simulink library "ptc"  (Simulink 8.1)
settings: Solver=ode1  StartTime=0.0  StopTime=Inf  FixedStep=0.001  RelTol=1e-3
PostLoadFcn:
  | , if any(exist('dsrtsu_mdlpostloadfcn', 'file') == [2, 3, 6]), try dsrtsu_mdlpostloadfcn('Execute', bdroot); catch fprintf('Error in PostLoadFcn (dsrtsu_mdlpostloadfcn) for model "%s":\n %s\n', bdroot, lasterr); end, end,
undefined symbols (not defined in the file or in its folder): AACC_ACCVehSpd_kph, MACC_ACCTorqueReq_Nm
libraries: simulink x3
settings Model: DSRTSU_INTERNAL_RTI_VER=450  DSRTSU_INTERNAL_RTI_TYPE=rti1401  RTICANMMDATA=struct('GeneralSetupData',struct('modelroot','D:\ELN150201_TAIWAN\trunk\AdasDragon\software\sw_development\arch\app\acc','generalsettings',struct('filesettings',struct('destfolder',struct('Name','RTICANMM_FILES','Check',1),'buildfolder',struct('Name','.','Check',1),'AbsDestfolder',struct('Name','D:\ELN150201_TAIWAN\trunk\AdasDragon\software\sw_development\arch\app\acc\RTICANMM_FILES'),'AbsBuildfolder',struct('Name','D:\ELN150201_TAIWAN\trunk\AdasDragon\software\sw_development\arch\app\acc'))),'options',struct('addpaths',1,'rmpaths',1,'addtrcexclusion',logical(1),'cannavigator',struct('checkmonitoring',0),'show_usrtrc',0,'use_usrtrc',0),'advanced',struct('options',[1 1 1 1 1 1 1 1 1 1 1 1 1 1 1 1 1 1 1 1 1 1 1 1 1 1 1 1 1 1 1 1 1 1 1 1 1 1 1 1 1 1 1 1 1 1 1 1 1 1 1 1 1 1 1 1 1 1 1 1 1 1 1 1 1 1 1 1 1 1 1 1 1 1 1 1 1 1 1 1 1 1 1 1 1 1 1 1 1 1 1 1 1 1 1 1 1 1 1 1]),'MPSetup',{{}},'modelname','ptc','block','ptc'))  DSRTSU_INTERNAL_RTIFPGA=40  Creator=AT015411  LastModifiedBy=AT015555

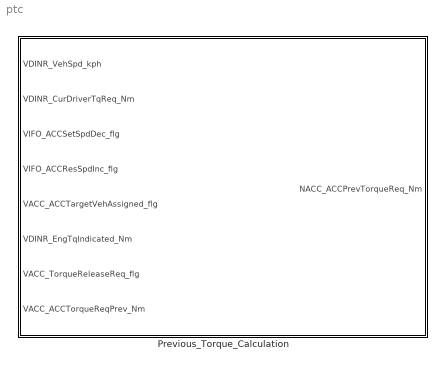
== system ptc ==
  Previous_Torque_Calculation : Subsystem

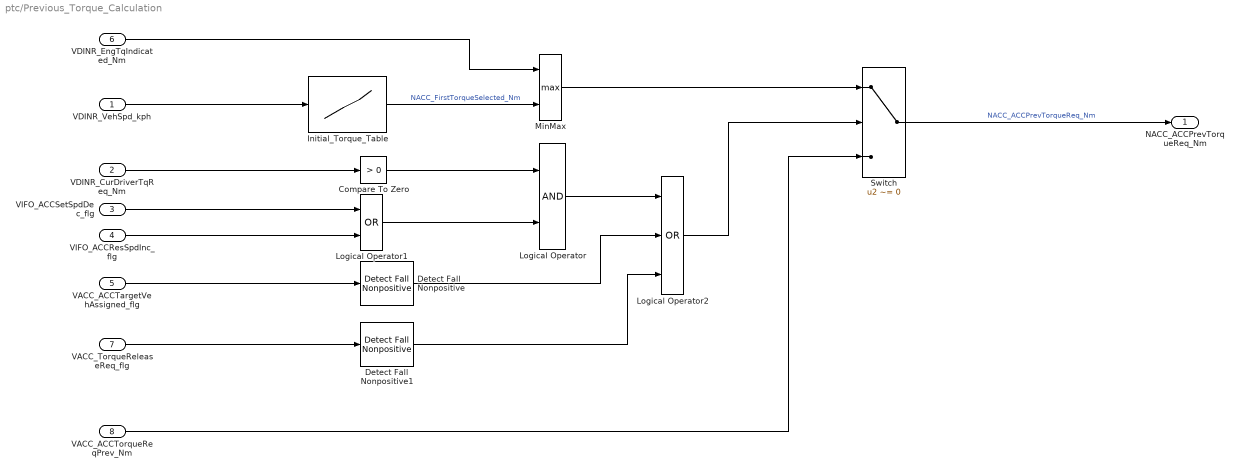
== system ptc/Previous_Torque_Calculation ==
  VDINR_VehSpd_kph : Inport
  VDINR_CurDriverTqReq_Nm : Inport  Port=2
  VIFO_ACCSetSpdDec_flg : Inport  Port=3
  VIFO_ACCResSpdInc_flg : Inport  Port=4
  VACC_ACCTargetVehAssigned_flg : Inport  Port=5
  VDINR_EngTqIndicated_Nm : Inport  Port=6
  VACC_TorqueReleaseReq_flg : Inport  Port=7
  VACC_ACCTorqueReqPrev_Nm : Inport  Port=8
  Compare To Zero : simulink/Logic and Bit Operations/Compare To Zero  relop=>  OutDataTypeStr=boolean
  Detect Fall Nonpositive : simulink/Logic and Bit Operations/Detect Fall Nonpositive  vinit=1  InputProcessing=Inherited  OutDataTypeStr=boolean
  Detect Fall Nonpositive1 : simulink/Logic and Bit Operations/Detect Fall Nonpositive  vinit=1  InputProcessing=Inherited  OutDataTypeStr=boolean
  Initial_Torque_Table : Lookup_n-D  NumberOfTableDimensions=1  BreakpointsForDimension1=AACC_ACCVehSpd_kph  Table=MACC_ACCTorqueReq_Nm  ExtrapMethod=Clip  UseLastTableValue=on  RndMeth=Simplest  InputSameDT=on
  Logical Operator : Logic  AllPortsSameDT=off  OutDataTypeStr=boolean
  Logical Operator1 : Logic  Operator=OR  AllPortsSameDT=off  OutDataTypeStr=boolean
  Logical Operator2 : Logic  Operator=OR  Inputs=3  AllPortsSameDT=off  OutDataTypeStr=boolean
  MinMax : MinMax  Function=max  Inputs=2
  Switch : Switch  Criteria=u2 ~= 0
  NACC_ACCPrevTorqueReq_Nm : Outport
  wires:
  Detect Fall Nonpositive/1 -> Logical Operator2/2
  VACC_ACCTargetVehAssigned_flg/1 -> Detect Fall Nonpositive/1
  Logical Operator/1 -> Logical Operator2/1
  Logical Operator2/1 -> Switch/2
  Logical Operator1/1 -> Logical Operator/2
  VIFO_ACCSetSpdDec_flg/1 -> Logical Operator1/1
  VIFO_ACCResSpdInc_flg/1 -> Logical Operator1/2
  VDINR_CurDriverTqReq_Nm/1 -> Compare To Zero/1
  Compare To Zero/1 -> Logical Operator/1
  Switch/1 -> NACC_ACCPrevTorqueReq_Nm/1  "NACC_ACCPrevTorqueReq_Nm"
  Initial_Torque_Table/1 -> MinMax/2  "NACC_FirstTorqueSelected_Nm"
  VDINR_VehSpd_kph/1 -> Initial_Torque_Table/1
  VACC_ACCTorqueReqPrev_Nm/1 -> Switch/3
  VDINR_EngTqIndicated_Nm/1 -> MinMax/1
  MinMax/1 -> Switch/1
  Detect Fall Nonpositive1/1 -> Logical Operator2/3
  VACC_TorqueReleaseReq_flg/1 -> Detect Fall Nonpositive1/1
